simulink model "mStateflowDSMBasicNameMapping"  (R2013b)
settings: Solver=FixedStepDiscrete  StartTime=0.0  StopTime=0.1  RelTol=1e-3
libraries: simulink x1
settings Model: Creator=hungdang  LastModifiedBy=hungdang
settings DataIOCC: SaveFormat=StructureWithTime
settings OptimizationCC: ActiveStateOutputEnumStorageType=Target Integer

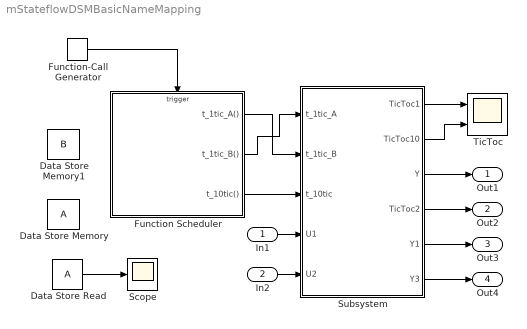
== system mStateflowDSMBasicNameMapping ==
  In1 : Inport  OutDataTypeStr=double  PortDimensions=1  SampleTime=0.001
  In2 : Inport  Port=2  OutDataTypeStr=double  PortDimensions=1  SampleTime=0.001
  Data Store Memory : DataStoreMemory  ReadBeforeWriteMsg=warning  WriteAfterWriteMsg=warning  WriteAfterReadMsg=warning  OutDataTypeStr=int8
  Data Store Memory1 : DataStoreMemory  DataStoreName=B  ReadBeforeWriteMsg=warning  WriteAfterWriteMsg=warning  WriteAfterReadMsg=warning  OutDataTypeStr=int8
  Data Store Read : DataStoreRead
  Function Scheduler : Stateflow chart  TreatAsAtomicUnit=on
  Function-Call Generator : simulink/Ports & Subsystems/Function-Call Generator  sample_time=0.001  numberOfIterations=1
  Scope : Scope
  Subsystem : Subsystem
  TicToc : Scope  NumInputPorts=2
      settings: TimeRange=0.025  YMin=0~-1  YMax=1~1
  Out1 : Outport
  Out2 : Outport  Port=2
  Out3 : Outport  Port=3
  Out4 : Outport  Port=4
  wires:
  Function-Call Generator/1 -> Function Scheduler/Trigger
  In1/1 -> Subsystem/4(U1)
  In2/1 -> Subsystem/5(U2)
  Subsystem/3(Y) -> Out1/1
  Function Scheduler/3(t_10tic()) -> Subsystem/3(t_10tic)
  Subsystem/1(TicToc1) -> TicToc/1
  Subsystem/2(TicToc10) -> TicToc/2
  Subsystem/4(TicToc2) -> Out2/1
  Function Scheduler/1(t_1tic_A()) -> Subsystem/2(t_1tic_B)
  Function Scheduler/2(t_1tic_B()) -> Subsystem/1(t_1tic_A)
  Data Store Read/1 -> Scope/1
  Subsystem/5(Y1) -> Out3/1
  Subsystem/6(Y3) -> Out4/1

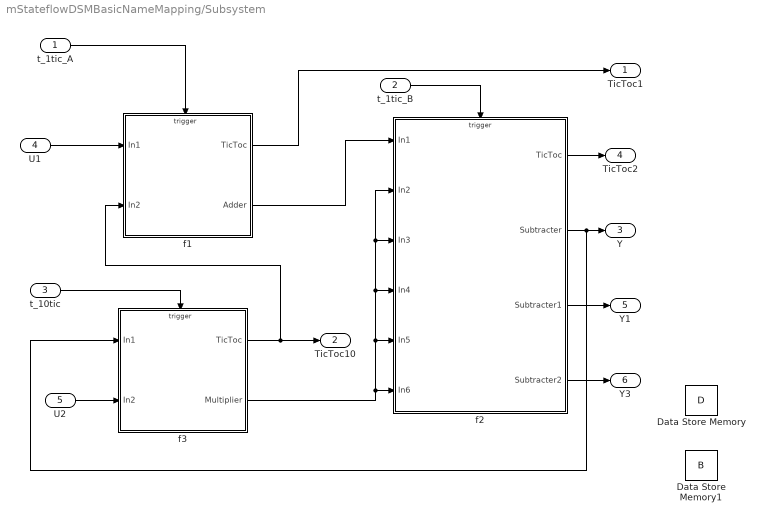
== system mStateflowDSMBasicNameMapping/Subsystem ==
  t_1tic_A : Inport
  t_1tic_B : Inport  Port=2
  t_10tic : Inport  Port=3
  U1 : Inport  Port=4
  U2 : Inport  Port=5
  Data Store Memory : DataStoreMemory  DataStoreName=D  ReadBeforeWriteMsg=warning  WriteAfterWriteMsg=warning  WriteAfterReadMsg=warning  OutDataTypeStr=int8
  Data Store Memory1 : DataStoreMemory  DataStoreName=B  ReadBeforeWriteMsg=warning  WriteAfterWriteMsg=warning  WriteAfterReadMsg=warning  OutDataTypeStr=int8
  f1 : Subsystem  TreatAsAtomicUnit=on  RTWFcnName=foo
  f2 : Subsystem  TreatAsAtomicUnit=on  RTWFcnName=foo
  f3 : Subsystem  TreatAsAtomicUnit=on  RTWFcnName=foo
  TicToc1 : Outport
  TicToc10 : Outport  Port=2
  Y : Outport  Port=3
  TicToc2 : Outport  Port=4
  Y1 : Outport  Port=5
  Y3 : Outport  Port=6
  wires:
  t_10tic/1 -> f3/Trigger
  U2/1 -> f3/2(In2)
  f2/2(Subtracter) -> Y/1, f3/1(In1)
  f1/2(Adder) -> f2/1(In1)
  f3/2(Multiplier) -> f2/6(In6), f2/4(In4), f2/3(In3), f2/2(In2), f2/5(In5)
  t_1tic_A/1 -> f1/Trigger
  f3/1(TicToc) -> f1/2(In2), TicToc10/1
  f2/1(TicToc) -> TicToc2/1
  f1/1(TicToc) -> TicToc1/1
  t_1tic_B/1 -> f2/Trigger
  U1/1 -> f1/1(In1)
  f2/3(Subtracter1) -> Y1/1
  f2/4(Subtracter2) -> Y3/1

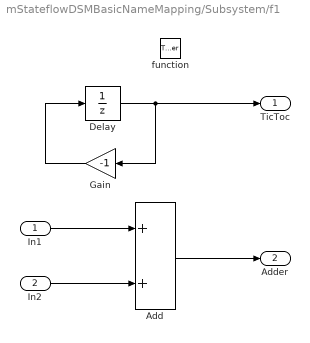
== system mStateflowDSMBasicNameMapping/Subsystem/f1 ==
  In1 : Inport
  In2 : Inport  Port=2
  function : TriggerPort  TriggerType=function-call
  Add : Sum
  Delay : UnitDelay  InitialCondition=1  SampleTime=-1
  Gain : Gain  Gain=-1  OutDataTypeStr=fixdt(1,8,0)
  TicToc : Outport  InitialOutput=0
  Adder : Outport  Port=2  InitialOutput=0
  wires:
  Add/1 -> Adder/1
  Gain/1 -> Delay/1
  Delay/1 -> TicToc/1, Gain/1
  In1/1 -> Add/1
  In2/1 -> Add/2

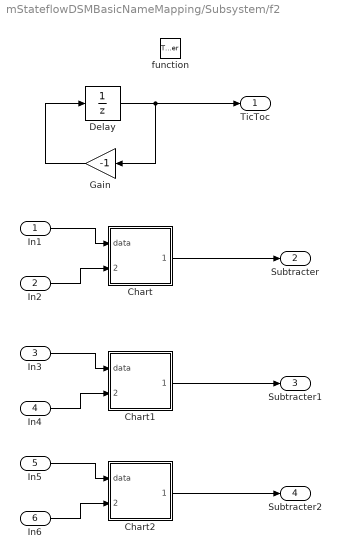
== system mStateflowDSMBasicNameMapping/Subsystem/f2 ==
  In1 : Inport
  In2 : Inport  Port=2
  In3 : Inport  Port=3
  In4 : Inport  Port=4
  In5 : Inport  Port=5
  In6 : Inport  Port=6
  function : TriggerPort  TriggerType=function-call
  Chart : Stateflow chart  TreatAsAtomicUnit=on
  Chart1 : Stateflow chart  TreatAsAtomicUnit=on
  Chart2 : Stateflow chart  TreatAsAtomicUnit=on
  Delay : UnitDelay  InitialCondition=1  SampleTime=-1
  Gain : Gain  Gain=-1  OutDataTypeStr=fixdt(1,8,0)
  TicToc : Outport  InitialOutput=0
  Subtracter : Outport  Port=2  InitialOutput=0
  Subtracter1 : Outport  Port=3  InitialOutput=0
  Subtracter2 : Outport  Port=4  InitialOutput=0
  wires:
  In2/1 -> Chart/2(data1)
  In1/1 -> Chart/1(data)
  Delay/1 -> Gain/1, TicToc/1
  Gain/1 -> Delay/1
  Chart/1(data2) -> Subtracter/1
  In4/1 -> Chart1/2(data1)
  In3/1 -> Chart1/1(data)
  Chart1/1(data2) -> Subtracter1/1
  In6/1 -> Chart2/2(data1)
  In5/1 -> Chart2/1(data)
  Chart2/1(data2) -> Subtracter2/1

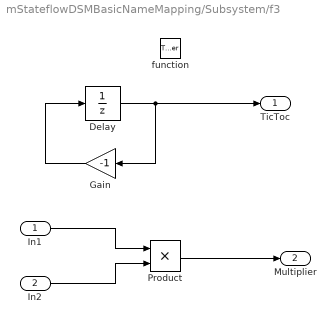
== system mStateflowDSMBasicNameMapping/Subsystem/f3 ==
  In1 : Inport
  In2 : Inport  Port=2
  function : TriggerPort  TriggerType=function-call
  Delay : UnitDelay  InitialCondition=1  SampleTime=-1
  Gain : Gain  Gain=-1  OutDataTypeStr=fixdt(1,8,0)
  Product : Product  Inputs=**  OutDataTypeStr=Inherit: Same as first input
  TicToc : Outport  InitialOutput=0
  Multiplier : Outport  Port=2  InitialOutput=0
  wires:
  In2/1 -> Product/2
  In1/1 -> Product/1
  Delay/1 -> Gain/1, TicToc/1
  Gain/1 -> Delay/1
  Product/1 -> Multiplier/1

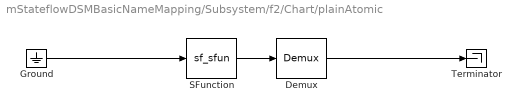
== system mStateflowDSMBasicNameMapping/Subsystem/f2/Chart/plainAtomic ==
  " Demux " : Demux  Outputs=1
  " Ground " : Ground
  " SFunction " : S-Function  Tag=Stateflow S-Function mStateflowDSMBasicNameMapping 5  FunctionName=sf_sfun  PortCounts=[1 1]  EnableBusSupport=off
  " Terminator " : Terminator
  wires:
  " Ground "/1 -> " SFunction "/1
  " Demux "/1 -> " Terminator "/1
  " SFunction "/1 -> " Demux "/1

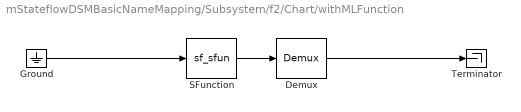
== system mStateflowDSMBasicNameMapping/Subsystem/f2/Chart/withMLFunction ==
  " Demux " : Demux  Outputs=1
  " Ground " : Ground
  " SFunction " : S-Function  Tag=Stateflow S-Function mStateflowDSMBasicNameMapping 6  FunctionName=sf_sfun  PortCounts=[1 1]  EnableBusSupport=off
  " Terminator " : Terminator
  wires:
  " Ground "/1 -> " SFunction "/1
  " Demux "/1 -> " Terminator "/1
  " SFunction "/1 -> " Demux "/1

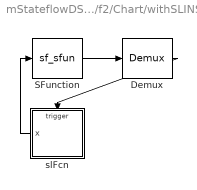
== system mStateflowDSMBasicNameMapping/Subsystem/f2/Chart/withSLINSF ==
  " Demux " : Demux  Outputs=1
  " SFunction " : S-Function  Tag=Stateflow S-Function mStateflowDSMBasicNameMapping 7  FunctionName=sf_sfun  PortCounts=[1 1]  EnableBusSupport=off
  slFcn : Subsystem
      settings: UndoDeleteFcn=Stateflow.SLINSF.SimulinkMan.restorePreDeleteFcn  PreDeleteFcn=Stateflow.SLINSF.SimulinkMan.removePreDeleteFcn
  wires:
  slFcn/1(x) -> " SFunction "/1
  " Demux "/1 -> slFcn/Trigger
  " SFunction "/1 -> " Demux "/1

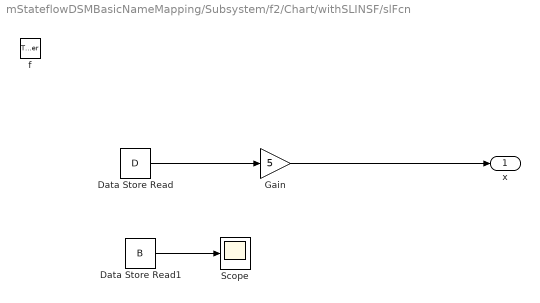
== system mStateflowDSMBasicNameMapping/Subsystem/f2/Chart/withSLINSF/slFcn ==
  f : TriggerPort  TriggerType=function-call
      settings: CopyFcn=Stateflow.SLINSF.SimulinkMan.removeBlockPreDeleteFcn  PreDeleteFcn=Stateflow.SLINSF.SimulinkMan.unsafePredeleteFcn
  Data Store Read : DataStoreRead  DataStoreName=D
  Data Store Read1 : DataStoreRead  DataStoreName=B
  Gain : Gain  Gain=5
  Scope : Scope
      settings: SaveName=ScopeData2
  x : Outport
  wires:
  Data Store Read/1 -> Gain/1
  Gain/1 -> x/1
  Data Store Read1/1 -> Scope/1

== stateflow chart mStateflowDSMBasicNameMapping/Function Scheduler ==
  settings: initializeOutput=1
  state OneTic [parallel]
    entry: t_1tic_B; t_1tic_A;
    on every(1,tic):
    t_1tic_B; t_1tic_A;
    settings: executionOrder=1
  state TenTic [parallel]
    entry: t_10tic;
    on every(10,tic): t_10tic;
    settings: executionOrder=2
  events: tic input FUNCTION_CALL_EVENT; t_1tic_A output FUNCTION_CALL_EVENT; t_1tic_B output FUNCTION_CALL_EVENT; t_10tic output FUNCTION_CALL_EVENT

== stateflow chart mStateflowDSMBasicNameMapping/Subsystem/f2/Chart ==
  state plainAtomic
  state withMLFunction
  state withSLINSF
  (default) -> plainAtomic : {data2 = data + data1 + A;}
  plainAtomic -> withMLFunction
  withMLFunction -> withSLINSF
  data: data input; data1 input; data2 output double; A data_store_memory

== stateflow chart mStateflowDSMBasicNameMapping/Subsystem/f2/Chart1 ==
  (default) -> (junction 6) : {data2 = data + data1 + A;}
  data: data input; data1 input; data2 output double; A data_store_memory

== stateflow chart mStateflowDSMBasicNameMapping/Subsystem/f2/Chart2 ==
  (default) -> (junction 6) : {A = data + data1;}
  data: data input; data1 input; data2 output double; A data_store_memory

== stateflow chart mStateflowDSMBasicNameMapping/Subsystem/f2/Chart/plainAtomic ==
  (default) -> (junction 3) : {ml.fprintf('%d\n', D);}
  data: D data_store_memory

== matlab function mStateflowDSMBasicNameMapping/Subsystem/f2/Chart/withMLFunction ==
  data: x function_output int8; D data_store_memory
function x = mlFunc
 
    x = D + int8(1);

== stateflow chart mStateflowDSMBasicNameMapping/Subsystem/f2/Chart/withSLINSF ==
  state x = slFcn [function]
  (default) -> (junction 3) : {ml.display(slFcn());}
  data: x function_output; D data_store_memory
